simulink model "ACMtr_180"  (R2019b)
settings: Solver=VariableStepAuto  StartTime=0.0  StopTime=0.04  RelTol=1e-3
settings Model: Creator=DELL  LastModifiedBy=DELL

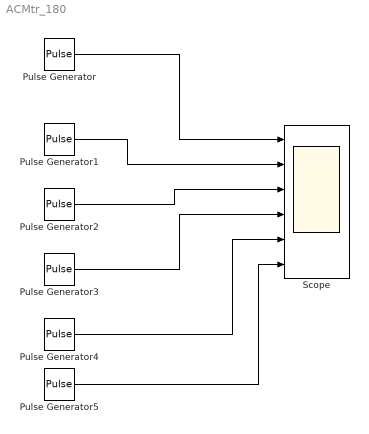
== system ACMtr_180 ==
  Pulse Generator : DiscretePulseGenerator  PulseType=Time based  Period=20e-3  PulseWidth=50
  Pulse Generator1 : DiscretePulseGenerator  PulseType=Time based  Period=20e-3  PulseWidth=50  PhaseDelay=20e-3/6
  Pulse Generator2 : DiscretePulseGenerator  PulseType=Time based  Period=20e-3  PulseWidth=50  PhaseDelay=2*(20e-3/6)
  Pulse Generator3 : DiscretePulseGenerator  PulseType=Time based  Period=20e-3  PulseWidth=50  PhaseDelay=3*(20e-3/6)
  Pulse Generator4 : DiscretePulseGenerator  PulseType=Time based  Period=20e-3  PulseWidth=50  PhaseDelay=4*(20e-3/6)
  Pulse Generator5 : DiscretePulseGenerator  PulseType=Time based  Period=20e-3  PulseWidth=50  PhaseDelay=5*(20e-3/6)
  Scope : Scope  NumInputPorts=6
  wires:
  Pulse Generator/1 -> Scope/1
  Pulse Generator1/1 -> Scope/2
  Pulse Generator2/1 -> Scope/3
  Pulse Generator3/1 -> Scope/4
  Pulse Generator4/1 -> Scope/5
  Pulse Generator5/1 -> Scope/6
